simulink model "rst_auto_reg_teste"  (R2019a)
settings: Solver=VariableStepAuto  StartTime=0.0  StopTime=500  RelTol=1e-3
values from neighbouring files (symbols this model uses):
  A = den    [cod_teste_RST_4.m]
  B = num    [cod_teste_RST_4.m]
  ep = 0.9    [cod_teste_RST_4.m]
  R = [X(5) X(6) X(7) X(8)]    [cod_teste_RST_4.m]
  S = [X(1) X(2) X(3) X(4)]    [cod_teste_RST_4.m]
  T = sum(Am)/sum(B)    [cod_teste_RST_4.m]
  Ta = 0.1    [cod_teste_RST_4.m]
  Ts = 1    [cod_teste_RST_4.m]
undefined symbols (not defined in the file or in its folder): T_a
libraries: dspinverses x3
settings Model: Creator=Carlos Henrique  LastModifiedBy=PICHAU
settings DataIOCC: SaveOutput=off  SaveState=on  SignalLogging=off  DSMLogging=off  ReturnWorkspaceOutputs=off
settings DebuggingCC: ArithmeticOperatorsInVariantConditions=warning

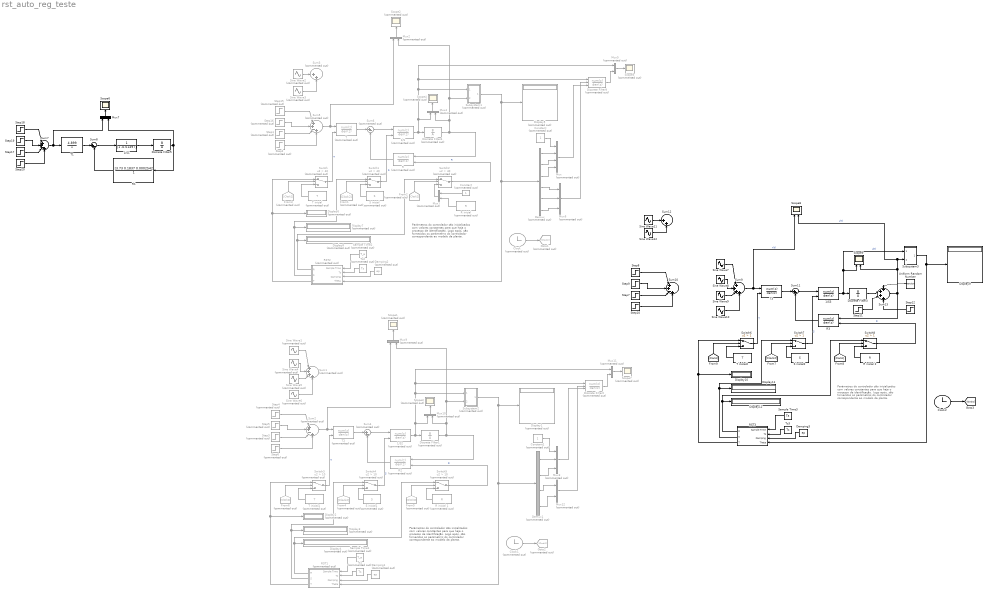
== system rst_auto_reg_teste ==
  note: Parâmetros do controlador são inicializados
      | com valores constantes para que haja o
      | processo de identificação. Logo após, são
      | fornecidos os parâmetros do controlador
      | correspondente ao modelo da planta.
  note: Parâmetros do controlador são inicializados
      | com valores constantes para que haja o
      | processo de identificação. Logo após, são
      | fornecidos os parâmetros do controlador
      | correspondente ao modelo da planta.
  note: Parâmetros do controlador são inicializados
      | com valores constantes para que haja o
      | processo de identificação. Logo após, são
      | fornecidos os parâmetros do controlador
      | correspondente ao modelo da planta.
  1/S : DiscreteFilter  Commented=on  Numerator=1  DenominatorSource=Input port  Denominator=1  a0EqualsOne=on
      settings: InputPortMap=u0,p3
  1/S1 : DiscreteFilter  Numerator=1  Denominator=[1 -0.01497]  a0EqualsOne=on
  1/S2 : DiscreteFilter  Commented=on  Numerator=1  DenominatorSource=Input port  Denominator=1  a0EqualsOne=on
      settings: InputPortMap=u0,p3
  1/S3 : DiscreteFilter  Numerator=1  DenominatorSource=Input port  Denominator=1  a0EqualsOne=on
      settings: InputPortMap=u0,p3
  Clock : Clock  Commented=on
  Clock1 : Clock  Commented=on
  Clock2 : Clock
  Constant : Constant  Commented=on
  "Constant " : Constant  Commented=on
  Constant1 : Constant  Commented=on
  Damping1 : Constant  Commented=on  Value=ep
  Damping2 : Constant  Commented=on  Value=ep
  Damping3 : Constant  Value=ep
  Demux : Demux  Commented=on  Outputs=6
  Demux1 : Demux  Commented=on
  Discrete Filter1 : DiscreteFilter  Commented=on  Numerator=B  Denominator=A  SampleTime=0.1  a0EqualsOne=on
  Discrete Filter2 : DiscreteFilter  Commented=on  NumeratorSource=Input port  Numerator=[3.317e-09 0.0355 0.02469]  DenominatorSource=Input port  Denominator=[1 -1.272 0.3317 0.0004192]  a0EqualsOne=on
      settings: InputPortMap=u0,p1,p3
  Discrete Filter3 : DiscreteFilter  Numerator=B  Denominator=A  SampleTime=0.1  a0EqualsOne=on
  Discrete Filter4 : DiscreteFilter  Commented=on  Numerator=B  Denominator=A  SampleTime=0.1  a0EqualsOne=on
  Discrete Filter5 : DiscreteFilter  Numerator=B  Denominator=A  SampleTime=0.1  a0EqualsOne=on
  Discrete Filter9 : DiscreteFilter  Commented=on  NumeratorSource=Input port  Numerator=[3.317e-09 0.0355 0.02469]  DenominatorSource=Input port  Denominator=[1 -1.272 0.3317 0.0004192]  a0EqualsOne=on
      settings: InputPortMap=u0,p1,p3
  Display{1..8} (8 alike) : Display  Commented=on
  Display{9..12} (4 alike) : Display
  From{1..6} (6 alike) : From  Commented=on  GotoTag=Clock2
  Goto1 : Goto  Commented=on  GotoTag=Clock2
  Goto2 : Goto  Commented=on  GotoTag=Clock2
  Mux : Mux  Commented=on
  Mux{1..2,4..5,9..12} (8 alike) : Mux  Commented=on  Inputs=2
  Mux3 : Mux  Commented=on  Inputs=3
  Mux6 : Mux  Commented=on  Inputs=3
  Mux7 : Mux  Inputs=2
  R : DiscreteFilter  Commented=on  NumeratorSource=Input port  Numerator=[-620.2 131.3]  Denominator=1
      settings: InputPortMap=u0,p1
  "R inicial " : Constant  Commented=on  Value=R
  R inicial 1 : Constant  Commented=on  Value=R
  R inicial 2 : Constant  Value=R
  R1 : DiscreteFilter  Numerator=[3.73 0.1837 0.0002542]  Denominator=1
  R2 : DiscreteFilter  Commented=on  NumeratorSource=Input port  Numerator=[-620.2 131.3]  Denominator=1
      settings: InputPortMap=u0,p1
  R3 : DiscreteFilter  NumeratorSource=Input port  Numerator=[-620.2 131.3]  Denominator=1
      settings: InputPortMap=u0,p1
  RST1 : Subsystem  Commented=on
  RST2 : Subsystem  Commented=on
  RST3 : Subsystem
  S inicial : Constant  Commented=on  Value=S
  S inicial1 : Constant  Commented=on  Value=S
  S inicial2 : Constant  Value=S
  Sample Time1 : Constant  Commented=on  Value=T_a
  Sample Time2 : Constant  Commented=on  Value=T_a
  Sample Time3 : Constant  Value=Ta
  Scope{1..5,7} (6 alike) : Scope  Commented=on
  Scope6 : Scope
  Scope8 : Scope  NumInputPorts=2
  Scope9 : Scope  NumInputPorts=2
  Sine Wave1 : Sin  Commented=on  SampleTime=0
  Sine Wave10 : Sin  Frequency=8  SampleTime=0
  Sine Wave11 : Sin  SampleTime=0
  Sine Wave12 : Sin  Frequency=2  SampleTime=0
  Sine Wave2 : Sin  Commented=on  SampleTime=0
  Sine Wave3 : Sin  Commented=on  Frequency=2  SampleTime=0
  Sine Wave4 : Sin  Commented=on  Frequency=2  SampleTime=0
  Sine Wave5 : Sin  Commented=on  Frequency=4  SampleTime=0
  Sine Wave6 : Sin  Commented=on  Frequency=8  SampleTime=0
  Sine Wave7 : Sin  SampleTime=0
  Sine Wave8 : Sin  Frequency=2  SampleTime=0
  Sine Wave9 : Sin  Frequency=4  SampleTime=0
  Step1 : Step  Commented=on  Time=20  After=2  SampleTime=0
  Step10 : Step  Time=30  SampleTime=0
  Step11 : Step  Time=50  SampleTime=0
  Step12 : Step  Time=51  After=-1  SampleTime=0
  Step15 : Step  Commented=on  Time=0  SampleTime=0
  Step16 : Step  Commented=on  Time=10  After=3  SampleTime=0
  Step17 : Step  Time=20  After=2  SampleTime=0
  Step18 : Step  Time=0  SampleTime=0
  Step19 : Step  Time=10  After=3  SampleTime=0
  Step2 : Step  Commented=on  Time=30  SampleTime=0
  Step20 : Step  Time=30  SampleTime=0
  Step3 : Step  Commented=on  Time=20  After=2  SampleTime=0
  Step4 : Step  Commented=on  Time=0  SampleTime=0
  Step5 : Step  Commented=on  Time=10  After=3  SampleTime=0
  Step6 : Step  Commented=on  Time=30  SampleTime=0
  Step7 : Step  Time=20  After=2  SampleTime=0
  Step8 : Step  Time=0  SampleTime=0
  Step9 : Step  Time=10  After=3  SampleTime=0
  Subsystem1 : Subsystem  Commented=on
  Subsystem2 : Subsystem  Commented=on
  Subsystem3 : Subsystem
  Sum1 : Sum  Commented=on  Inputs=|++++
  Sum10 : Sum  Inputs=|++-+
  Sum11 : Sum  Inputs=|+-
  Sum12 : Sum  Inputs=|++
  Sum13 : Sum  Inputs=++++
  Sum2 : Sum  Commented=on  Inputs=|++-+
  Sum3 : Sum  Commented=on  Inputs=|++
  Sum4 : Sum  Commented=on  Inputs=|+-
  Sum5 : Sum  Commented=on  Inputs=|++-+
  Sum6 : Sum  Commented=on  Inputs=|+-
  Sum7 : Sum  Inputs=|++-+
  Sum8 : Sum  Inputs=|+-
  Sum9 : Sum  Inputs=|++++
  Switch : Switch  Commented=on  Criteria=u2 > Threshold  Threshold=40
  Switch1 : Switch  Commented=on  Criteria=u2 > Threshold  Threshold=40
  Switch2 : Switch  Commented=on  Criteria=u2 > Threshold  Threshold=40
  Switch3 : Switch  Commented=on  Criteria=u2 > Threshold  Threshold=10
  Switch4 : Switch  Commented=on  Criteria=u2 > Threshold  Threshold=10
  Switch5 : Switch  Commented=on  Criteria=u2 > Threshold  Threshold=10
  Switch6 : Switch  Criteria=u2 > Threshold  Threshold=1
  Switch7 : Switch  Criteria=u2 > Threshold  Threshold=1
  Switch8 : Switch  Criteria=u2 > Threshold  Threshold=1
  T : DiscreteFilter  Commented=on  NumeratorSource=Input port  Numerator=13.39  Denominator=1
      settings: InputPortMap=u0,p1
  T inicial : Constant  Commented=on  Value=T
  T inicial1 : Constant  Commented=on  Value=T
  T inicial2 : Constant  Value=T
  T1 : DiscreteFilter  Numerator=4.899  Denominator=1  a0EqualsOne=on
  T2 : DiscreteFilter  Commented=on  NumeratorSource=Input port  Numerator=13.39  Denominator=1
      settings: InputPortMap=u0,p1
  T3 : DiscreteFilter  NumeratorSource=Input port  Numerator=13.39  Denominator=1
      settings: InputPortMap=u0,p1
  Ts1 : Constant  Commented=on  Value=Ts
  Ts2 : Constant  Commented=on  Value=Ts
  Ts3 : Constant  Value=Ts
  Uniform Random Number : UniformRandomNumber  Minimum=-0.1  Maximum=0.1  SampleTime=0
  wires:
  Sum6/1 -> 1/S/1
  R/1 -> Sum6/2
  Ts2/1 -> RST2/2(Ts)
  Step2/1 -> Sum5/4
  Damping2/1 -> RST2/3(Damping)
  Sum5/1 -> Mux2/1, T/1
  T/1 -> Sum6/1
  Step1/1 -> Sum5/3
  Step15/1 -> Sum5/1
  Step16/1 -> Sum5/2
  RST2/3(T) -> Switch/1, Display6/1
  Sample Time2/1 -> RST2/1(Sample Time)
  RST2/2(S) -> Switch1/1, Display7/1
  Mux5/1 -> Scope5/1
  Constant/1 -> Mux/1
  Demux/1 -> Mux/2
  Demux/2 -> Mux/3
  Demux/3 -> Mux/4
  Demux/4 -> Mux6/1
  Demux/5 -> Mux6/2
  Demux/6 -> Mux6/3
  Mux/1 -> Discrete Filter9/3
  Mux6/1 -> Discrete Filter9/2
  Discrete Filter9/1 -> Mux5/2
  1/S/1 -> Mux5/1, Discrete Filter9/1, Subsystem1/1(In1), Mux4/1, Discrete Filter4/1
  RST2/1(R) -> Switch2/1, Display8/1
  1/S1/1 -> Discrete Filter5/1
  Discrete Filter5/1 -> R1/1, Mux7/2
  Mux7/1 -> Scope6/1
  Step19/1 -> Sum7/2
  Step18/1 -> Sum7/1
  Step17/1 -> Sum7/3
  T1/1 -> Sum8/1
  Sum7/1 -> Mux7/1, T1/1
  Step20/1 -> Sum7/4
  R1/1 -> Sum8/2
  Sum8/1 -> 1/S1/1
  Discrete Filter4/1 -> R/1, Subsystem1/2(In2), Mux2/2, Mux4/2
  Mux4/1 -> Scope4/1
  T inicial/1 -> Switch/3
  From3/1 -> Switch/2
  Clock/1 -> Goto1/1
  Switch/1 -> T/2  "T"
  From1/1 -> Switch1/2
  Switch1/1 -> 1/S/2  "S"
  From2/1 -> Switch2/2
  Switch2/1 -> R/2  "R"
  S inicial/1 -> Switch1/3
  "R inicial "/1 -> Mux1/2
  "Constant "/1 -> Mux1/1
  Mux1/1 -> Switch2/3
  Subsystem1/1(Out1) -> RST2/4(Theta), Demux/1, Display5/1
  Mux2/1 -> Scope2/1
  Sine Wave2/1 -> Sum3/1
  Sine Wave3/1 -> Sum3/2
  Sine Wave4/1 -> Sum1/2
  Switch3/1 -> T2/2  "T"
  Mux9/1 -> Scope1/1
  Subsystem2/1(Out1) -> RST1/4(Theta), Demux1/1, Display1/1
  Switch4/1 -> 1/S2/2  "S"
  Switch5/1 -> R2/2  "R"
  Sum2/1 -> Mux9/1, T2/1
  Discrete Filter1/1 -> R2/1, Subsystem2/2(In2), Mux9/2, Mux10/2
  S inicial1/1 -> Switch4/3
  Sine Wave1/1 -> Sum1/1
  RST1/3(T) -> Switch3/1, Display2/1
  Damping1/1 -> RST1/3(Damping)
  T inicial1/1 -> Switch3/3
  From4/1 -> Switch4/2
  Sum4/1 -> 1/S2/1
  Mux10/1 -> Scope3/1
  Step5/1 -> Sum2/2
  Clock1/1 -> Goto2/1
  From6/1 -> Switch3/2
  From5/1 -> Switch5/2
  Demux1/1 -> Mux3/2
  Discrete Filter2/1 -> Mux11/2
  RST1/1(R) -> Switch5/1, Display4/1
  Mux3/1 -> Discrete Filter2/3
  1/S2/1 -> Mux11/1, Discrete Filter2/1, Subsystem2/1(In1), Mux10/1, Discrete Filter1/1
  Demux1/2 -> Mux3/3
  Mux11/1 -> Scope7/1
  Constant1/1 -> Mux3/1
  Step4/1 -> Sum2/1
  Mux12/1 -> Discrete Filter2/2
  Sample Time1/1 -> RST1/1(Sample Time)
  Step3/1 -> Sum2/3
  Step6/1 -> Sum2/4
  RST1/2(S) -> Switch4/1, Display3/1
  Ts1/1 -> RST1/2(Ts)
  R2/1 -> Sum4/2
  T2/1 -> Sum4/1
  Demux1/3 -> Mux12/1
  Demux1/4 -> Mux12/2
  R inicial 1/1 -> Switch5/3
  Sine Wave5/1 -> Sum1/3
  Sine Wave6/1 -> Sum1/4
  Sine Wave10/1 -> Sum9/4
  Ts3/1 -> RST3/2(Ts)
  T3/1 -> Sum11/1
  R3/1 -> Sum11/2
  RST3/1(R) -> Switch8/1, Display12/1
  Switch8/1 -> R3/2  "R"
  Step7/1 -> Sum10/3
  RST3/2(S) -> Switch7/1, Display11/1
  [Clock2] -> Switch7/2
  Sum13/1 -> R3/1, Scope9/2, Subsystem3/2(In2), Scope8/2  "y(t)"
  Subsystem3/1(Out1) -> RST3/4(Theta), Display9/1
  T inicial2/1 -> Switch6/3
  Sine Wave7/1 -> Sum9/1
  Clock2/1 -> [Clock2]
  S inicial2/1 -> Switch7/3
  Sum11/1 -> 1/S3/1
  Switch6/1 -> T3/2  "T"
  [Clock2] -> Switch6/2
  Switch7/1 -> 1/S3/2  "S"
  Sample Time3/1 -> RST3/1(Sample Time)
  Sine Wave8/1 -> Sum9/2
  Damping3/1 -> RST3/3(Damping)
  RST3/3(T) -> Switch6/1, Display10/1
  R inicial 2/1 -> Switch8/3
  Sine Wave9/1 -> Sum9/3
  Step9/1 -> Sum10/2
  Step8/1 -> Sum10/1
  Step10/1 -> Sum10/4
  1/S3/1 -> Scope9/1, Subsystem3/1(In1), Discrete Filter3/1  "u(t)"
  [Clock2] -> Switch8/2
  Sine Wave12/1 -> Sum12/2
  Sine Wave11/1 -> Sum12/1
  Discrete Filter3/1 -> Sum13/2
  Uniform Random Number/1 -> Sum13/1
  Step11/1 -> Sum13/3
  Step12/1 -> Sum13/4
  Sum9/1 -> Scope8/1, T3/1  "r(t)"

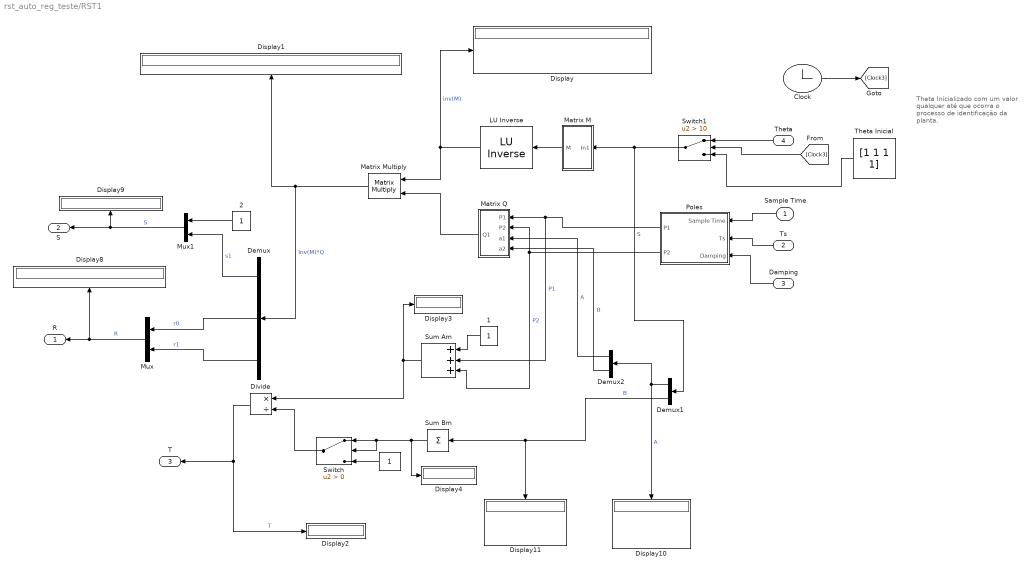
== system rst_auto_reg_teste/RST1 ==
  note: Theta Inicializado com um
      | valor qualquer até que ocorra
      |  o processo de identificação
      | da planta.
  Sample Time : Inport
  Ts : Inport  Port=2
  Damping : Inport  Port=3
  Theta : Inport  Port=4
  " " : Constant
  " LU Inverse" : dspinverses/ LU Inverse
      settings: SourceProductName=DSP System Toolbox
  1 : Constant
  2 : Constant
  Clock : Clock
  Demux : Demux  Outputs=3
  Demux1 : Demux  Outputs=2
  Demux2 : Demux  Outputs=2
  Display{,1..4,8..11} (9 alike) : Display
  Divide : Product  Inputs=*/
  Matrix M : Subsystem
  Matrix Multiply : Product  Multiplication=Matrix(*)
  Matrix Q : Subsystem
  Mux : Mux  Inputs=2
  Mux1 : Mux  Inputs=2
  Poles : Subsystem
  Sum Am : Sum  Inputs=+++
  Sum Bm : Sum  Inputs=+
  Switch : Switch  Criteria=u2 > Threshold
  Switch1 : Switch  Criteria=u2 > Threshold  Threshold=10
  Theta Inicial : Constant  Value=[1 1 1 1]
  R : Outport
  S : Outport  Port=2
  T : Outport  Port=3
  wires:
  Matrix Multiply/1 -> Demux/1, Display1/1  "Inv(M)*Q"
  Sum Bm/1 -> Switch/2, Switch/1, Display4/1
  " LU Inverse"/1 -> Matrix Multiply/1, Display/1  "inv(M)"
  Sum Am/1 -> Divide/1, Display3/1
  Mux1/1 -> S/1, Display9/1  "S"
  Poles/2(P2) -> Sum Am/3, Matrix Q/2(P2)  "P2"
  Divide/1 -> T/1, Display2/1  "T"
  Ts/1 -> Poles/2(Ts)
  Damping/1 -> Poles/3(Damping)
  Sample Time/1 -> Poles/1(Sample Time)
  1/1 -> Sum Am/1
  Poles/1(P1) -> Sum Am/2, Matrix Q/1(P1)  "P1"
  Demux1/2 -> Display11/1, Sum Bm/1  "B"
  Demux1/1 -> Display10/1, Demux2/1  "A"
  Switch/1 -> Divide/2
  " "/1 -> Switch/3
  Mux/1 -> R/1, Display8/1  "R"
  Clock/1 -> [Clock3]
  Switch1/1 -> Matrix M/1(In1), Demux1/1  "S"
  Theta/1 -> Switch1/1
  [Clock3] -> Switch1/2
  Theta Inicial/1 -> Switch1/3
  Matrix M/1(M) -> " LU Inverse"/1
  Matrix Q/1(Q1) -> Matrix Multiply/2
  Demux2/1 -> Matrix Q/3(a1)  "A"
  Demux2/2 -> Matrix Q/4(a2)  "B"
  Demux/2 -> Mux/1  "r0"
  Demux/3 -> Mux/2  "r1"
  Demux/1 -> Mux1/2  "s1"
  2/1 -> Mux1/1

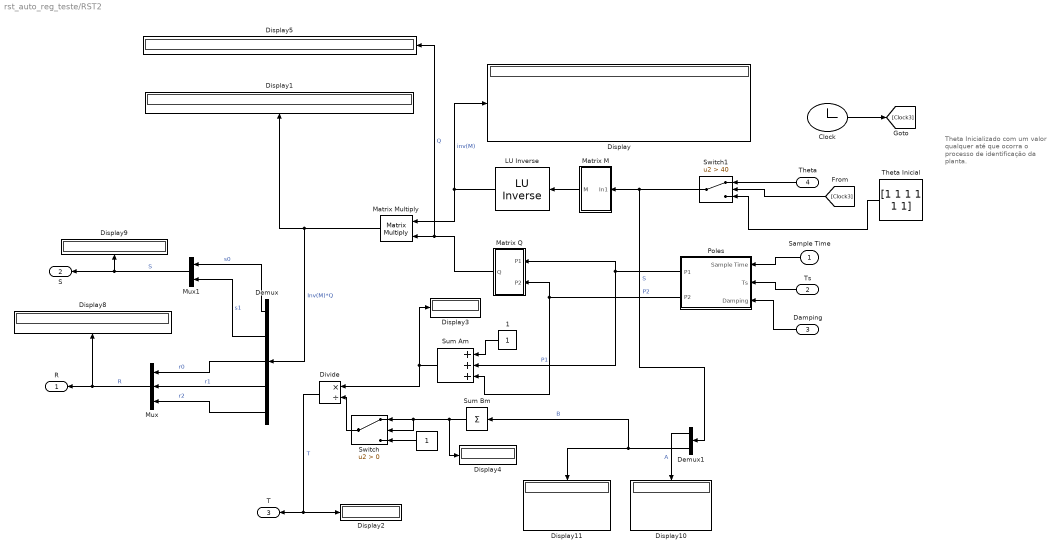
== system rst_auto_reg_teste/RST2 ==
  note: Theta Inicializado com um
      | valor qualquer até que ocorra
      |  o processo de identificação
      | da planta.
  Sample Time : Inport
  Ts : Inport  Port=2
  Damping : Inport  Port=3
  Theta : Inport  Port=4
  " " : Constant
  " LU Inverse" : dspinverses/ LU Inverse
      settings: SourceProductName=DSP System Toolbox
  1 : Constant
  Clock : Clock
  Demux : Demux  Outputs=5
  Demux1 : Demux  Outputs=2
  Display{,1..5,8..11} (10 alike) : Display
  Divide : Product  Inputs=*/
  Matrix M : Subsystem
  Matrix Multiply : Product  Multiplication=Matrix(*)
  Matrix Q : Subsystem
  Mux : Mux  Inputs=3
  Mux1 : Mux  Inputs=2
  Poles : Subsystem
  Sum Am : Sum  Inputs=+++
  Sum Bm : Sum  Inputs=+
  Switch : Switch  Criteria=u2 > Threshold
  Switch1 : Switch  Criteria=u2 > Threshold  Threshold=40
  Theta Inicial : Constant  Value=[1 1 1 1 1 1]
  R : Outport
  S : Outport  Port=2
  T : Outport  Port=3
  wires:
  Matrix Multiply/1 -> Demux/1, Display1/1  "Inv(M)*Q"
  Sum Bm/1 -> Switch/2, Switch/1, Display4/1
  " LU Inverse"/1 -> Matrix Multiply/1, Display/1  "inv(M)"
  Sum Am/1 -> Divide/1, Display3/1
  Mux1/1 -> S/1, Display9/1  "S"
  Poles/2(P2) -> Matrix Q/2(P2), Sum Am/3  "P2"
  Divide/1 -> T/1, Display2/1  "T"
  Ts/1 -> Poles/2(Ts)
  Matrix Q/1(Q) -> Display5/1, Matrix Multiply/2  "Q"
  Damping/1 -> Poles/3(Damping)
  Sample Time/1 -> Poles/1(Sample Time)
  1/1 -> Sum Am/1
  Matrix M/1(M) -> " LU Inverse"/1
  Poles/1(P1) -> Sum Am/2, Matrix Q/1(P1)  "P1"
  Demux1/2 -> Sum Bm/1, Display11/1  "B"
  Demux1/1 -> Display10/1  "A"
  Switch/1 -> Divide/2
  " "/1 -> Switch/3
  Demux/1 -> Mux1/1  "s0"
  Demux/2 -> Mux1/2  "s1"
  Mux/1 -> R/1, Display8/1  "R"
  Demux/3 -> Mux/1  "r0"
  Demux/4 -> Mux/2  "r1"
  Demux/5 -> Mux/3  "r2"
  Clock/1 -> [Clock3]
  Switch1/1 -> Demux1/1, Matrix M/1(In1)  "S"
  Theta/1 -> Switch1/1
  [Clock3] -> Switch1/2
  Theta Inicial/1 -> Switch1/3

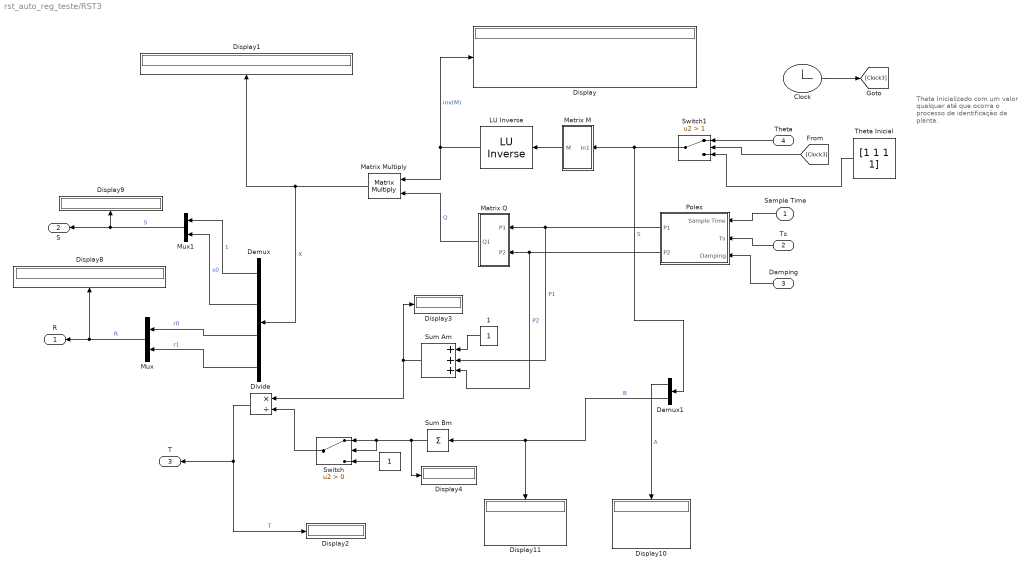
== system rst_auto_reg_teste/RST3 ==
  note: Theta Inicializado com um
      | valor qualquer até que ocorra
      |  o processo de identificação
      | da planta.
  Sample Time : Inport
  Ts : Inport  Port=2
  Damping : Inport  Port=3
  Theta : Inport  Port=4
  " " : Constant
  " LU Inverse" : dspinverses/ LU Inverse
      settings: SourceProductName=DSP System Toolbox
  1 : Constant
  Clock : Clock
  Demux : Demux
  Demux1 : Demux  Outputs=2
  Display{,1..4,8..11} (9 alike) : Display
  Divide : Product  Inputs=*/
  Matrix M : Subsystem
  Matrix Multiply : Product  Multiplication=Matrix(*)
  Matrix Q : Subsystem
  Mux : Mux  Inputs=2
  Mux1 : Mux  Inputs=2
  Poles : Subsystem
  Sum Am : Sum  Inputs=+++
  Sum Bm : Sum  Inputs=+
  Switch : Switch  Criteria=u2 > Threshold
  Switch1 : Switch  Criteria=u2 > Threshold  Threshold=1
  Theta Inicial : Constant  Value=[1 1 1 1]
  R : Outport
  S : Outport  Port=2
  T : Outport  Port=3
  wires:
  Matrix Multiply/1 -> Demux/1, Display1/1  "X"
  Sum Bm/1 -> Switch/2, Switch/1, Display4/1
  " LU Inverse"/1 -> Matrix Multiply/1, Display/1  "inv(M)"
  Sum Am/1 -> Divide/1, Display3/1
  Mux1/1 -> S/1, Display9/1  "S"
  Poles/2(P2) -> Matrix Q/2(P2), Sum Am/3  "P2"
  Divide/1 -> T/1, Display2/1  "T"
  Ts/1 -> Poles/2(Ts)
  Damping/1 -> Poles/3(Damping)
  Sample Time/1 -> Poles/1(Sample Time)
  1/1 -> Sum Am/1
  Poles/1(P1) -> Matrix Q/1(P1), Sum Am/2  "P1"
  Demux1/2 -> Display11/1, Sum Bm/1  "B"
  Demux1/1 -> Display10/1  "A"
  Switch/1 -> Divide/2
  " "/1 -> Switch/3
  Mux/1 -> R/1, Display8/1  "R"
  Clock/1 -> [Clock3]
  Switch1/1 -> Matrix M/1(In1), Demux1/1  "S"
  Theta/1 -> Switch1/1
  [Clock3] -> Switch1/2
  Theta Inicial/1 -> Switch1/3
  Matrix M/1(M) -> " LU Inverse"/1
  Matrix Q/1(Q1) -> Matrix Multiply/2  "Q"
  Demux/1 -> Mux1/1  "1"
  Demux/2 -> Mux1/2  "s0"
  Demux/3 -> Mux/1  "r0"
  Demux/4 -> Mux/2  "r1"

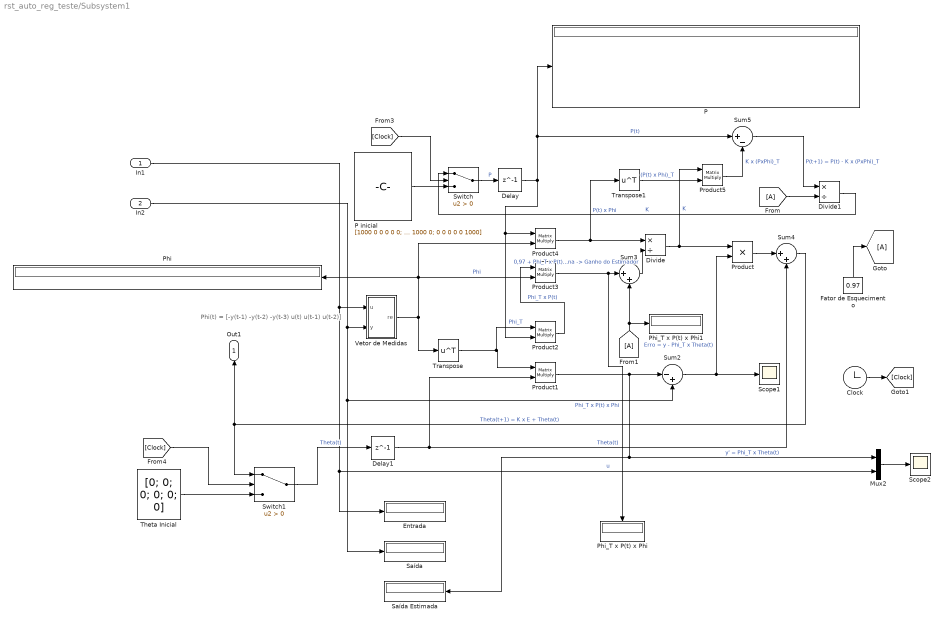
== system rst_auto_reg_teste/Subsystem1 ==
  note: Phi(t) = [-y(t-1) -y(t-2) -y(t-3) u(t) u(t-1) u(t-2)]
  In1 : Inport
  In2 : Inport  Port=2
  Clock : Clock
  Delay : Delay  DelayLength=1  InitialCondition=0  SampleTime=0.1
  Delay1 : Delay  DelayLength=1  InitialCondition=0  SampleTime=0.1
  Divide : Product  Inputs=*/
  Divide1 : Product  Inputs=*/
  Entrada : Display
  "Fator de Esquecimento " : Constant  Value=0.97
  Mux2 : Mux  Inputs=2
  P : Display
  P inicial : Constant  Value=[1000 0 0 0 0 0; 0 1000 0 0 0 0; 0 0 1000 0 0 0; 0 0 0 1000 0 0; 0 0 0 0 1000 0; 0 0 0 0 0 1000]
  Phi : Display
  Phi_T x P(t) x Phi : Display
  Phi_T x P(t) x Phi1 : Display
  Product : Product
  Product{1..5} (5 alike) : Product  Multiplication=Matrix(*)
  Saída : Display
  "Saída Estimada " : Display
  Scope1 : Scope
  Scope2 : Scope
  Sum2 : Sum  Inputs=|-+
  Sum3 : Sum  Inputs=|++
  Sum4 : Sum  Inputs=|++
  Sum5 : Sum  Inputs=|+-
  Switch : Switch  Criteria=u2 > Threshold
  Switch1 : Switch  Criteria=u2 > Threshold
  "Theta Inicial " : Constant  Value=[0; 0; 0; 0; 0; 0]
  Transpose : Math  Operator=transpose  SaturateOnIntegerOverflow=on
  Transpose1 : Math  Operator=transpose  SaturateOnIntegerOverflow=on
  "Vetor de Medidas " : Subsystem
  Out1 : Outport
  wires:
  "Vetor de Medidas "/1(re) -> Product4/2, Phi/1, Product3/2, Transpose/1  "Phi"
  Product/1 -> Sum4/1
  In2/1 -> Saída/1, Sum2/2, "Vetor de Medidas "/2(y)
  "Fator de Esquecimento "/1 -> [A]
  Transpose/1 -> Product2/1, Product1/1  "Phi_T"
  Sum3/1 -> Divide/2  "0,97 + Phi_T x P(t) x Phi Vetor Coluna -> Ganho do Estimador"
  Product3/1 -> Phi_T x P(t) x Phi/1, Sum3/1  "Phi_T x P(t) x Phi"
  Switch/1 -> Delay/1  "P"
  Product4/1 -> Transpose1/1, Divide/1  "P(t) x Phi"
  Delay/1 -> Product2/2, Product4/1, P/1, Sum5/1  "P(t)"
  Divide/1 -> Product5/1, Product/1  "K"
  Transpose1/1 -> Product5/2  "(P(t) x Phi)_T"
  Sum5/1 -> Divide1/1  "P(t+1) = P(t) - K x (PxPhi)_T"
  Sum2/1 -> Scope1/1, Product/2  "Erro = y - Phi_T x Theta(t)"
  Delay1/1 -> Sum4/2, Product1/2  "Theta(t)"
  Divide1/1 -> Switch/1  "K"
  "Theta Inicial "/1 -> Switch1/3
  [A] -> Divide1/2
  Product2/1 -> Product3/1  "Phi_T x P(t)"
  Clock/1 -> [Clock]
  Product1/1 -> Mux2/1, "Saída Estimada "/1, Sum2/1  "y' = Phi_T x Theta(t)"
  Product5/1 -> Sum5/2  "K x (PxPhi)_T"
  P inicial/1 -> Switch/3
  Sum4/1 -> Switch1/1, Out1/1  "Theta(t+1) = K x E + Theta(t)"
  [A] -> Sum3/2, Phi_T x P(t) x Phi1/1
  In1/1 -> Entrada/1, Mux2/2, "Vetor de Medidas "/1(u)  "u"
  [Clock] -> Switch/2
  Switch1/1 -> Delay1/1  "Theta(t)"
  Mux2/1 -> Scope2/1
  [Clock] -> Switch1/2

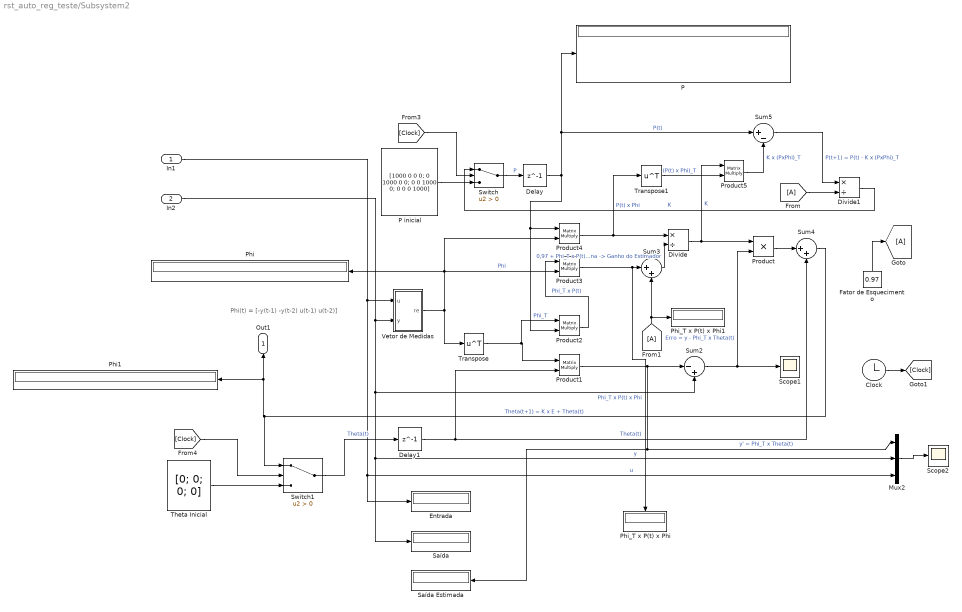
== system rst_auto_reg_teste/Subsystem2 ==
  note: Phi(t) = [-y(t-1) -y(t-2) u(t-1) u(t-2)]
  In1 : Inport
  In2 : Inport  Port=2
  Clock : Clock
  Delay : Delay  DelayLength=1  InitialCondition=0  SampleTime=0.1
  Delay1 : Delay  DelayLength=1  InitialCondition=0  SampleTime=0.1
  Divide : Product  Inputs=*/
  Divide1 : Product  Inputs=*/
  Entrada : Display
  "Fator de Esquecimento " : Constant  Value=0.97
  Mux2 : Mux  Inputs=3
  P : Display
  P inicial : Constant  Value=[1000 0 0 0; 0 1000 0 0; 0 0 1000 0; 0 0 0 1000]
  Phi : Display
  Phi1 : Display
  Phi_T x P(t) x Phi : Display
  Phi_T x P(t) x Phi1 : Display
  Product : Product
  Product{1..5} (5 alike) : Product  Multiplication=Matrix(*)
  Saída : Display
  "Saída Estimada " : Display
  Scope1 : Scope
  Scope2 : Scope
  Sum2 : Sum  Inputs=|-+
  Sum3 : Sum  Inputs=|++
  Sum4 : Sum  Inputs=|++
  Sum5 : Sum  Inputs=|+-
  Switch : Switch  Criteria=u2 > Threshold
  Switch1 : Switch  Criteria=u2 > Threshold
  "Theta Inicial " : Constant  Value=[0; 0; 0; 0]
  Transpose : Math  Operator=transpose  SaturateOnIntegerOverflow=on
  Transpose1 : Math  Operator=transpose  SaturateOnIntegerOverflow=on
  "Vetor de Medidas " : Subsystem
  Out1 : Outport
  wires:
  "Vetor de Medidas "/1(re) -> Product4/2, Phi/1, Product3/2, Transpose/1  "Phi"
  Product/1 -> Sum4/1
  In2/1 -> Mux2/2, Saída/1, Sum2/2, "Vetor de Medidas "/2(y)  "y"
  "Fator de Esquecimento "/1 -> [A]
  Transpose/1 -> Product2/1, Product1/1  "Phi_T"
  Sum3/1 -> Divide/2  "0,97 + Phi_T x P(t) x Phi Vetor Coluna -> Ganho do Estimador"
  Product3/1 -> Phi_T x P(t) x Phi/1, Sum3/1  "Phi_T x P(t) x Phi"
  Switch/1 -> Delay/1  "P"
  Product4/1 -> Transpose1/1, Divide/1  "P(t) x Phi"
  Delay/1 -> Product2/2, Product4/1, P/1, Sum5/1  "P(t)"
  Divide/1 -> Product5/1, Product/1  "K"
  Transpose1/1 -> Product5/2  "(P(t) x Phi)_T"
  Sum5/1 -> Divide1/1  "P(t+1) = P(t) - K x (PxPhi)_T"
  Sum2/1 -> Scope1/1, Product/2  "Erro = y - Phi_T x Theta(t)"
  Delay1/1 -> Sum4/2, Product1/2  "Theta(t)"
  Divide1/1 -> Switch/1  "K"
  "Theta Inicial "/1 -> Switch1/3
  [A] -> Divide1/2
  Product2/1 -> Product3/1  "Phi_T x P(t)"
  Clock/1 -> [Clock]
  Product1/1 -> Sum2/1, Mux2/1, "Saída Estimada "/1  "y' = Phi_T x Theta(t)"
  Product5/1 -> Sum5/2  "K x (PxPhi)_T"
  P inicial/1 -> Switch/3
  Sum4/1 -> Switch1/1, Phi1/1, Out1/1  "Theta(t+1) = K x E + Theta(t)"
  [A] -> Sum3/2, Phi_T x P(t) x Phi1/1
  In1/1 -> Mux2/3, Entrada/1, "Vetor de Medidas "/1(u)  "u"
  [Clock] -> Switch/2
  Switch1/1 -> Delay1/1  "Theta(t)"
  Mux2/1 -> Scope2/1
  [Clock] -> Switch1/2

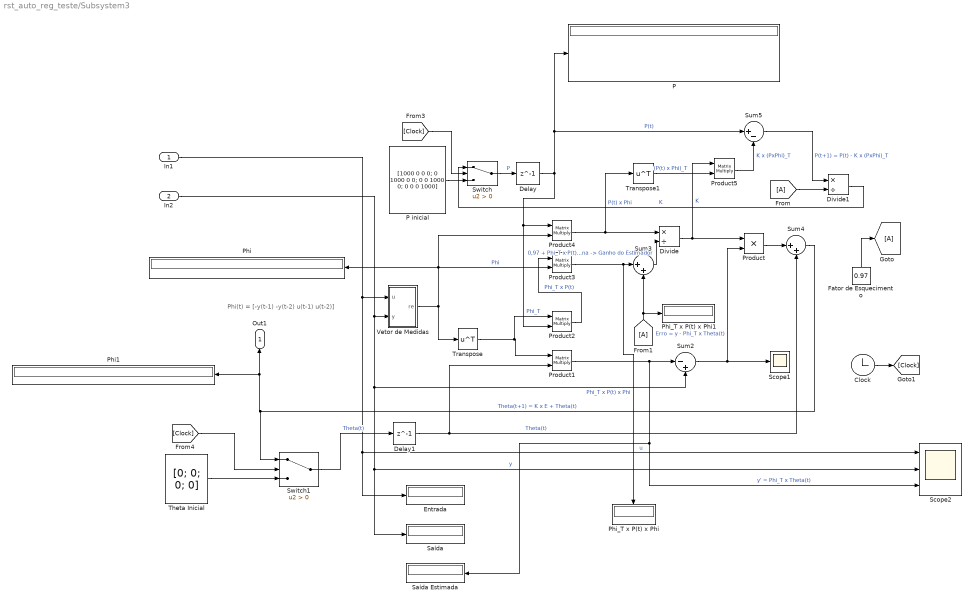
== system rst_auto_reg_teste/Subsystem3 ==
  note: Phi(t) = [-y(t-1) -y(t-2) u(t-1) u(t-2)]
  In1 : Inport
  In2 : Inport  Port=2
  Clock : Clock
  Delay : Delay  DelayLength=1  InitialCondition=0  SampleTime=0.1
  Delay1 : Delay  DelayLength=1  InitialCondition=0  SampleTime=0.1
  Divide : Product  Inputs=*/
  Divide1 : Product  Inputs=*/
  Entrada : Display
  "Fator de Esquecimento " : Constant  Value=0.97
  P : Display
  P inicial : Constant  Value=[1000 0 0 0; 0 1000 0 0; 0 0 1000 0; 0 0 0 1000]
  Phi : Display
  Phi1 : Display
  Phi_T x P(t) x Phi : Display
  Phi_T x P(t) x Phi1 : Display
  Product : Product
  Product{1..5} (5 alike) : Product  Multiplication=Matrix(*)
  Saída : Display
  "Saída Estimada " : Display
  Scope1 : Scope
  Scope2 : Scope  NumInputPorts=3
  Sum2 : Sum  Inputs=|-+
  Sum3 : Sum  Inputs=|++
  Sum4 : Sum  Inputs=|++
  Sum5 : Sum  Inputs=|+-
  Switch : Switch  Criteria=u2 > Threshold
  Switch1 : Switch  Criteria=u2 > Threshold
  "Theta Inicial " : Constant  Value=[0; 0; 0; 0]
  Transpose : Math  Operator=transpose  SaturateOnIntegerOverflow=on
  Transpose1 : Math  Operator=transpose  SaturateOnIntegerOverflow=on
  "Vetor de Medidas " : Subsystem
  Out1 : Outport
  wires:
  "Vetor de Medidas "/1(re) -> Product4/2, Phi/1, Product3/2, Transpose/1  "Phi"
  Product/1 -> Sum4/1
  In2/1 -> Saída/1, Scope2/2, Sum2/2, "Vetor de Medidas "/2(y)  "y"
  "Fator de Esquecimento "/1 -> [A]
  Transpose/1 -> Product2/1, Product1/1  "Phi_T"
  Sum3/1 -> Divide/2  "0,97 + Phi_T x P(t) x Phi Vetor Coluna -> Ganho do Estimador"
  Product3/1 -> Phi_T x P(t) x Phi/1, Sum3/1  "Phi_T x P(t) x Phi"
  Switch/1 -> Delay/1  "P"
  Product4/1 -> Transpose1/1, Divide/1  "P(t) x Phi"
  Delay/1 -> Product2/2, Product4/1, P/1, Sum5/1  "P(t)"
  Divide/1 -> Product5/1, Product/1  "K"
  Transpose1/1 -> Product5/2  "(P(t) x Phi)_T"
  Sum5/1 -> Divide1/1  "P(t+1) = P(t) - K x (PxPhi)_T"
  Sum2/1 -> Scope1/1, Product/2  "Erro = y - Phi_T x Theta(t)"
  Delay1/1 -> Sum4/2, Product1/2  "Theta(t)"
  Divide1/1 -> Switch/1  "K"
  "Theta Inicial "/1 -> Switch1/3
  [A] -> Divide1/2
  Product2/1 -> Product3/1  "Phi_T x P(t)"
  Clock/1 -> [Clock]
  Product1/1 -> Sum2/1, Scope2/3, "Saída Estimada "/1  "y' = Phi_T x Theta(t)"
  Product5/1 -> Sum5/2  "K x (PxPhi)_T"
  P inicial/1 -> Switch/3
  Sum4/1 -> Switch1/1, Phi1/1, Out1/1  "Theta(t+1) = K x E + Theta(t)"
  [A] -> Sum3/2, Phi_T x P(t) x Phi1/1
  In1/1 -> Entrada/1, Scope2/1, "Vetor de Medidas "/1(u)  "u"
  [Clock] -> Switch/2
  Switch1/1 -> Delay1/1  "Theta(t)"
  [Clock] -> Switch1/2

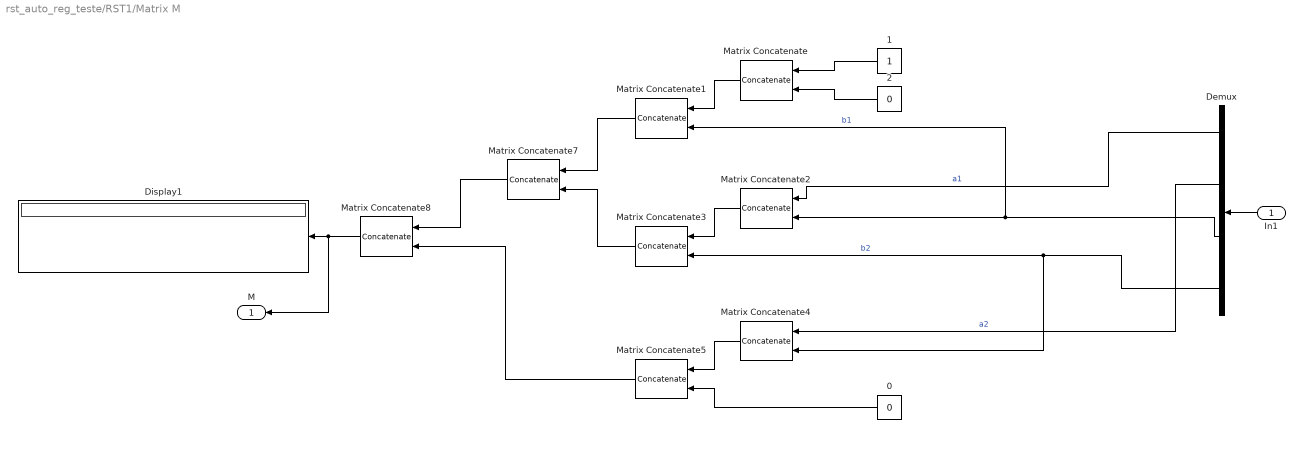
== system rst_auto_reg_teste/RST1/Matrix M ==
  In1 : Inport
  " 0" : Constant  Value=0
  " 2" : Constant  Value=0
  1 : Constant
  Demux : Demux
  Display1 : Display
  Matrix Concatenate{,1..5} (6 alike) : Concatenate  Mode=Multidimensional array  ConcatenateDimension=2
  Matrix Concatenate7 : Concatenate  Mode=Multidimensional array
  Matrix Concatenate8 : Concatenate  Mode=Multidimensional array
  M : Outport
  wires:
  In1/1 -> Demux/1
  1/1 -> Matrix Concatenate/1
  Matrix Concatenate5/1 -> Matrix Concatenate8/2
  Matrix Concatenate4/1 -> Matrix Concatenate5/1
  " 2"/1 -> Matrix Concatenate/2
  Demux/3 -> Matrix Concatenate1/2, Matrix Concatenate2/2  "b1"
  Matrix Concatenate2/1 -> Matrix Concatenate3/1
  Matrix Concatenate1/1 -> Matrix Concatenate7/1
  Matrix Concatenate3/1 -> Matrix Concatenate7/2
  " 0"/1 -> Matrix Concatenate5/2
  Matrix Concatenate7/1 -> Matrix Concatenate8/1
  Matrix Concatenate/1 -> Matrix Concatenate1/1
  Matrix Concatenate8/1 -> M/1, Display1/1
  Demux/1 -> Matrix Concatenate2/1  "a1"
  Demux/4 -> Matrix Concatenate4/2, Matrix Concatenate3/2  "b2"
  Demux/2 -> Matrix Concatenate4/1  "a2"

== system rst_auto_reg_teste/RST1/Matrix Q ==
  P1 : Inport
  P2 : Inport  Port=2
  a1 : Inport  Port=3
  a2 : Inport  Port=4
  2 : Constant  Value=0
  Display1 : Display
  Matrix Concatenate1 : Concatenate  Mode=Multidimensional array
  Matrix Concatenate2 : Concatenate  Mode=Multidimensional array
  Subtract : Sum  Inputs=+-
  Subtract1 : Sum  Inputs=+-
  Q1 : Outport
  wires:
  Subtract/1 -> Matrix Concatenate1/1
  P2/1 -> Subtract1/1
  Matrix Concatenate1/1 -> Matrix Concatenate2/1
  Matrix Concatenate2/1 -> Q1/1, Display1/1
  2/1 -> Matrix Concatenate2/2
  P1/1 -> Subtract/1
  Subtract1/1 -> Matrix Concatenate1/2
  a2/1 -> Subtract1/2
  a1/1 -> Subtract/2

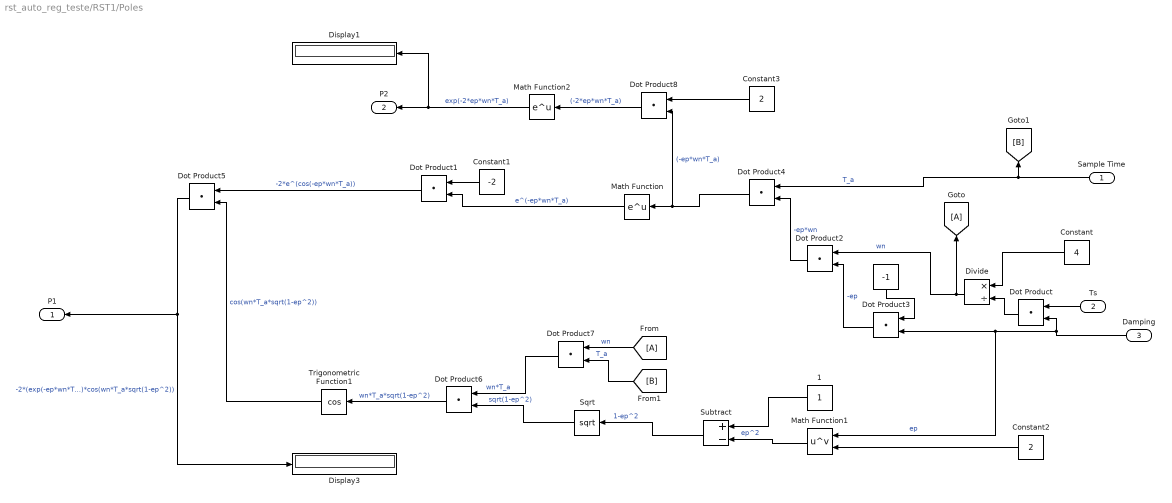
== system rst_auto_reg_teste/RST1/Poles ==
  Sample Time : Inport
  Ts : Inport  Port=2
  Damping : Inport  Port=3
  " " : Constant  Value=-1
  1 : Constant
  Constant : Constant  Value=4
  Constant1 : Constant  Value=-2
  Constant2 : Constant  Value=2
  Constant3 : Constant  Value=2
  Display1 : Display
  Display3 : Display
  Divide : Product  Inputs=*/
  Dot Product{,1..8} (9 alike) : DotProduct  InputSameDT=on  OutDataTypeStr=Inherit: Inherit via internal rule
  Math Function : Math  SaturateOnIntegerOverflow=on
  Math Function1 : Math  Operator=pow  SaturateOnIntegerOverflow=on
  Math Function2 : Math  SaturateOnIntegerOverflow=on
  Sqrt : Sqrt  SaturateOnIntegerOverflow=on
  Subtract : Sum  Inputs=+-
  Trigonometric Function1 : Trigonometry  Operator=cos
  P1 : Outport
  P2 : Outport  Port=2
  wires:
  Math Function/1 -> Dot Product1/2  "e^(-ep*wn*T_a)"
  Divide/1 -> [A], Dot Product2/1  "wn"
  [A] -> Dot Product7/1  "wn"
  " "/1 -> Dot Product3/1
  Dot Product5/1 -> P1/1, Display3/1  "-2*(exp(-ep*wn*T_a))*cos(wn*T_a*sqrt(1-ep^2))"
  Trigonometric Function1/1 -> Dot Product5/2  "cos(wn*T_a*sqrt(1-ep^2))"
  Ts/1 -> Dot Product/1
  Dot Product/1 -> Divide/2
  Dot Product3/1 -> Dot Product2/2  "-ep"
  Damping/1 -> Math Function1/1, Dot Product3/2, Dot Product/2  "ep"
  Constant/1 -> Divide/1
  Dot Product7/1 -> Dot Product6/1  "wn*T_a"
  Sample Time/1 -> Dot Product4/1, [B]  "T_a"
  Math Function1/1 -> Subtract/2  "ep^2"
  Dot Product1/1 -> Dot Product5/1  "-2*e^(cos(-ep*wn*T_a))"
  Constant2/1 -> Math Function1/2
  1/1 -> Subtract/1
  Constant1/1 -> Dot Product1/1
  Dot Product2/1 -> Dot Product4/2  "-ep*wn"
  [B] -> Dot Product7/2  "T_a"
  Dot Product6/1 -> Trigonometric Function1/1  "wn*T_a*sqrt(1-ep^2)"
  Dot Product4/1 -> Dot Product8/2, Math Function/1  "(-ep*wn*T_a)"
  Sqrt/1 -> Dot Product6/2  "sqrt(1-ep^2)"
  Subtract/1 -> Sqrt/1  "1-ep^2"
  Constant3/1 -> Dot Product8/1
  Dot Product8/1 -> Math Function2/1  "(-2*ep*wn*T_a)"
  Math Function2/1 -> Display1/1, P2/1  "exp(-2*ep*wn*T_a)"

== system rst_auto_reg_teste/RST2/Matrix M ==
  In1 : Inport
  " " : Constant  Value=0
  " 1" : Constant
  Demux : Demux  Outputs=6
  Display : Display
  Matrix Concatenate{,1..4} (5 alike) : Concatenate  NumInputs=5  Mode=Multidimensional array  ConcatenateDimension=2
  Matrix Concatenate6 : Concatenate  NumInputs=5  Mode=Multidimensional array
  M : Outport
  wires:
  In1/1 -> Demux/1
  Matrix Concatenate6/1 -> M/1, Display/1
  Matrix Concatenate/1 -> Matrix Concatenate6/1
  Matrix Concatenate2/1 -> Matrix Concatenate6/2
  Matrix Concatenate1/1 -> Matrix Concatenate6/3
  Matrix Concatenate3/1 -> Matrix Concatenate6/4
  " 1"/1 -> Matrix Concatenate2/2, Matrix Concatenate/1
  " "/1 -> Matrix Concatenate4/4, Matrix Concatenate4/3, Matrix Concatenate4/1, Matrix Concatenate3/3, Matrix Concatenate2/5, Matrix Concatenate/5, Matrix Concatenate/4, Matrix Concatenate/2
  Demux/4 -> Matrix Concatenate2/4, Matrix Concatenate/3, Matrix Concatenate1/5  "b0"
  Demux/1 -> Matrix Concatenate1/2, Matrix Concatenate2/1  "a1"
  Demux/5 -> Matrix Concatenate3/5, Matrix Concatenate1/4, Matrix Concatenate2/3  "b1"
  Demux/2 -> Matrix Concatenate3/2, Matrix Concatenate1/1  "a2"
  Demux/6 -> Matrix Concatenate4/5, Matrix Concatenate3/4, Matrix Concatenate1/3  "b2"
  Demux/3 -> Matrix Concatenate3/1, Matrix Concatenate4/2  "a3"
  Matrix Concatenate4/1 -> Matrix Concatenate6/5

== system rst_auto_reg_teste/RST2/Matrix Q ==
  P1 : Inport
  P2 : Inport  Port=2
  0 : Constant  Value=0
  1 : Constant
  Display : Display
  Matrix Concatenate : Concatenate  NumInputs=5  Mode=Multidimensional array
  Q : Outport
  wires:
  Matrix Concatenate/1 -> Q/1, Display/1
  1/1 -> Matrix Concatenate/1
  P1/1 -> Matrix Concatenate/2
  P2/1 -> Matrix Concatenate/3
  0/1 -> Matrix Concatenate/5, Matrix Concatenate/4

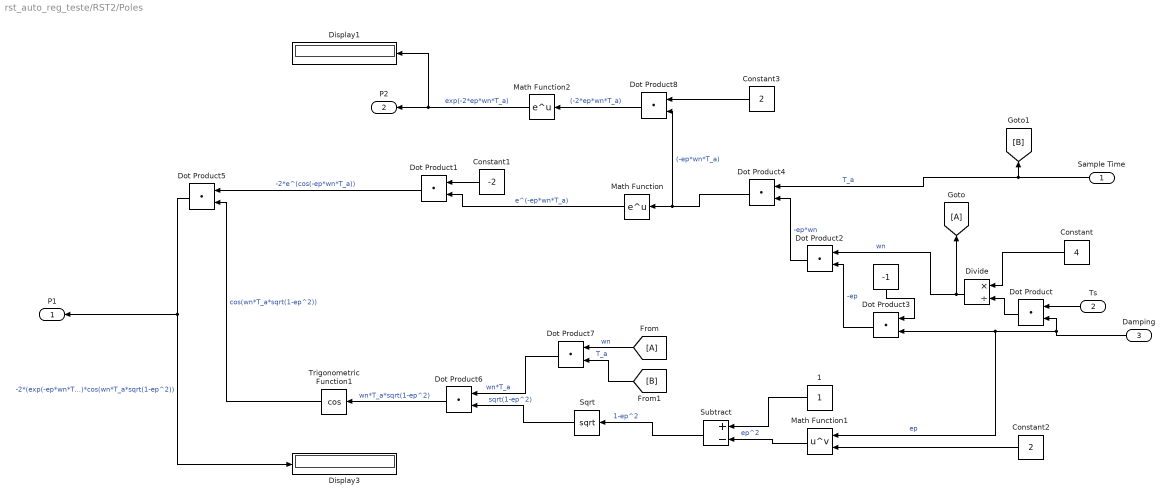
== system rst_auto_reg_teste/RST2/Poles ==
  Sample Time : Inport
  Ts : Inport  Port=2
  Damping : Inport  Port=3
  " " : Constant  Value=-1
  1 : Constant
  Constant : Constant  Value=4
  Constant1 : Constant  Value=-2
  Constant2 : Constant  Value=2
  Constant3 : Constant  Value=2
  Display1 : Display
  Display3 : Display
  Divide : Product  Inputs=*/
  Dot Product{,1..8} (9 alike) : DotProduct  InputSameDT=on  OutDataTypeStr=Inherit: Inherit via internal rule
  Math Function : Math  SaturateOnIntegerOverflow=on
  Math Function1 : Math  Operator=pow  SaturateOnIntegerOverflow=on
  Math Function2 : Math  SaturateOnIntegerOverflow=on
  Sqrt : Sqrt  SaturateOnIntegerOverflow=on
  Subtract : Sum  Inputs=+-
  Trigonometric Function1 : Trigonometry  Operator=cos
  P1 : Outport
  P2 : Outport  Port=2
  wires:
  Math Function/1 -> Dot Product1/2  "e^(-ep*wn*T_a)"
  Divide/1 -> [A], Dot Product2/1  "wn"
  [A] -> Dot Product7/1  "wn"
  " "/1 -> Dot Product3/1
  Dot Product5/1 -> P1/1, Display3/1  "-2*(exp(-ep*wn*T_a))*cos(wn*T_a*sqrt(1-ep^2))"
  Trigonometric Function1/1 -> Dot Product5/2  "cos(wn*T_a*sqrt(1-ep^2))"
  Ts/1 -> Dot Product/1
  Dot Product/1 -> Divide/2
  Dot Product3/1 -> Dot Product2/2  "-ep"
  Damping/1 -> Math Function1/1, Dot Product3/2, Dot Product/2  "ep"
  Constant/1 -> Divide/1
  Dot Product7/1 -> Dot Product6/1  "wn*T_a"
  Sample Time/1 -> Dot Product4/1, [B]  "T_a"
  Math Function1/1 -> Subtract/2  "ep^2"
  Dot Product1/1 -> Dot Product5/1  "-2*e^(cos(-ep*wn*T_a))"
  Constant2/1 -> Math Function1/2
  1/1 -> Subtract/1
  Constant1/1 -> Dot Product1/1
  Dot Product2/1 -> Dot Product4/2  "-ep*wn"
  [B] -> Dot Product7/2  "T_a"
  Dot Product6/1 -> Trigonometric Function1/1  "wn*T_a*sqrt(1-ep^2)"
  Dot Product4/1 -> Dot Product8/2, Math Function/1  "(-ep*wn*T_a)"
  Sqrt/1 -> Dot Product6/2  "sqrt(1-ep^2)"
  Subtract/1 -> Sqrt/1  "1-ep^2"
  Constant3/1 -> Dot Product8/1
  Dot Product8/1 -> Math Function2/1  "(-2*ep*wn*T_a)"
  Math Function2/1 -> Display1/1, P2/1  "exp(-2*ep*wn*T_a)"

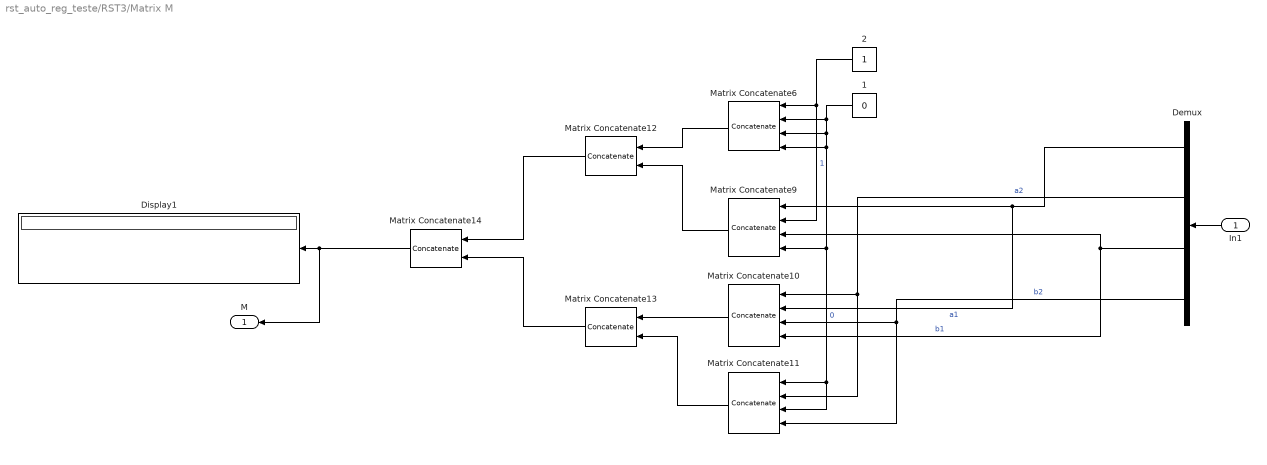
== system rst_auto_reg_teste/RST3/Matrix M ==
  In1 : Inport
  " 1" : Constant  Value=0
  2 : Constant
  Demux : Demux
  Display1 : Display
  Matrix Concatenate{6,9..11} (4 alike) : Concatenate  NumInputs=4  Mode=Multidimensional array  ConcatenateDimension=2
  Matrix Concatenate12 : Concatenate  Mode=Multidimensional array
  Matrix Concatenate13 : Concatenate  Mode=Multidimensional array
  Matrix Concatenate14 : Concatenate  Mode=Multidimensional array
  M : Outport
  wires:
  In1/1 -> Demux/1
  Demux/3 -> Matrix Concatenate9/3, Matrix Concatenate10/4  "b1"
  Matrix Concatenate14/1 -> M/1, Display1/1
  Demux/1 -> Matrix Concatenate10/2, Matrix Concatenate9/1  "a1"
  Demux/4 -> Matrix Concatenate11/4, Matrix Concatenate10/3  "b2"
  Demux/2 -> Matrix Concatenate11/2, Matrix Concatenate10/1  "a2"
  2/1 -> Matrix Concatenate9/2, Matrix Concatenate6/1  "1"
  " 1"/1 -> Matrix Concatenate6/3, Matrix Concatenate11/3, Matrix Concatenate11/1, Matrix Concatenate9/4, Matrix Concatenate6/4, Matrix Concatenate6/2  "0"
  Matrix Concatenate6/1 -> Matrix Concatenate12/1
  Matrix Concatenate9/1 -> Matrix Concatenate12/2
  Matrix Concatenate10/1 -> Matrix Concatenate13/1
  Matrix Concatenate11/1 -> Matrix Concatenate13/2
  Matrix Concatenate13/1 -> Matrix Concatenate14/2
  Matrix Concatenate12/1 -> Matrix Concatenate14/1

== system rst_auto_reg_teste/RST3/Matrix Q ==
  P1 : Inport
  P2 : Inport  Port=2
  Constant : Constant
  Constant1 : Constant  Value=0
  Display1 : Display
  Matrix Concatenate1 : Concatenate  Mode=Multidimensional array
  Matrix Concatenate2 : Concatenate  Mode=Multidimensional array
  Matrix Concatenate3 : Concatenate  Mode=Multidimensional array
  Q1 : Outport
  wires:
  Matrix Concatenate1/1 -> Matrix Concatenate2/1
  Matrix Concatenate2/1 -> Q1/1, Display1/1
  Matrix Concatenate3/1 -> Matrix Concatenate2/2
  P2/1 -> Matrix Concatenate3/1
  P1/1 -> Matrix Concatenate1/2
  Constant/1 -> Matrix Concatenate1/1
  Constant1/1 -> Matrix Concatenate3/2

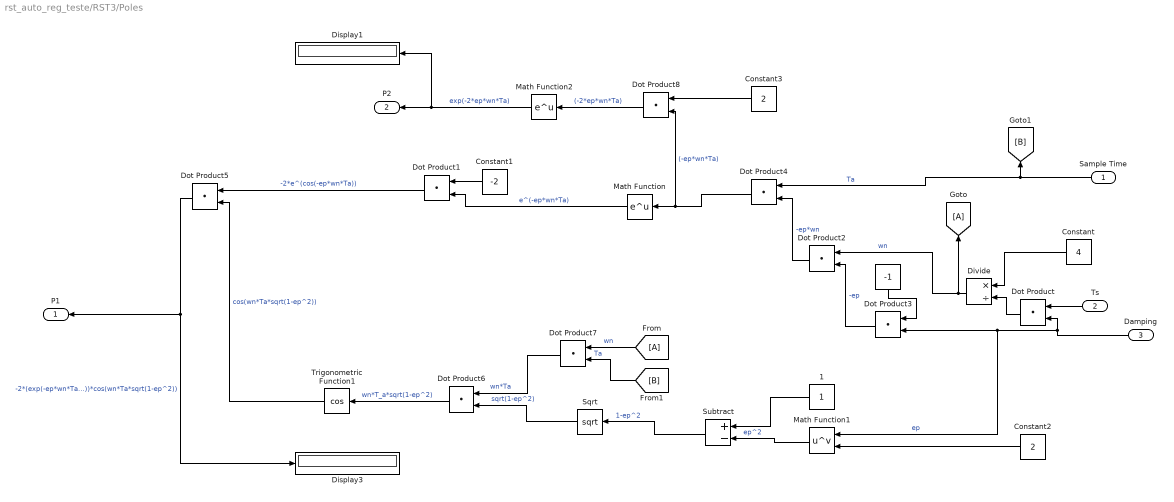
== system rst_auto_reg_teste/RST3/Poles ==
  Sample Time : Inport
  Ts : Inport  Port=2
  Damping : Inport  Port=3
  " " : Constant  Value=-1
  1 : Constant
  Constant : Constant  Value=4
  Constant1 : Constant  Value=-2
  Constant2 : Constant  Value=2
  Constant3 : Constant  Value=2
  Display1 : Display
  Display3 : Display
  Divide : Product  Inputs=*/
  Dot Product{,1..8} (9 alike) : DotProduct  InputSameDT=on  OutDataTypeStr=Inherit: Inherit via internal rule
  Math Function : Math  SaturateOnIntegerOverflow=on
  Math Function1 : Math  Operator=pow  SaturateOnIntegerOverflow=on
  Math Function2 : Math  SaturateOnIntegerOverflow=on
  Sqrt : Sqrt  SaturateOnIntegerOverflow=on
  Subtract : Sum  Inputs=+-
  Trigonometric Function1 : Trigonometry  Operator=cos
  P1 : Outport
  P2 : Outport  Port=2
  wires:
  Math Function/1 -> Dot Product1/2  "e^(-ep*wn*Ta)"
  Divide/1 -> [A], Dot Product2/1  "wn"
  [A] -> Dot Product7/1  "wn"
  " "/1 -> Dot Product3/1
  Dot Product5/1 -> P1/1, Display3/1  "-2*(exp(-ep*wn*Ta))*cos(wn*Ta*sqrt(1-ep^2))"
  Trigonometric Function1/1 -> Dot Product5/2  "cos(wn*Ta*sqrt(1-ep^2))"
  Ts/1 -> Dot Product/1
  Dot Product/1 -> Divide/2
  Dot Product3/1 -> Dot Product2/2  "-ep"
  Damping/1 -> Math Function1/1, Dot Product3/2, Dot Product/2  "ep"
  Constant/1 -> Divide/1
  Dot Product7/1 -> Dot Product6/1  "wn*Ta"
  Sample Time/1 -> Dot Product4/1, [B]  "Ta"
  Math Function1/1 -> Subtract/2  "ep^2"
  Dot Product1/1 -> Dot Product5/1  "-2*e^(cos(-ep*wn*Ta))"
  Constant2/1 -> Math Function1/2
  1/1 -> Subtract/1
  Constant1/1 -> Dot Product1/1
  Dot Product2/1 -> Dot Product4/2  "-ep*wn"
  [B] -> Dot Product7/2  "Ta"
  Dot Product6/1 -> Trigonometric Function1/1  "wn*T_a*sqrt(1-ep^2)"
  Dot Product4/1 -> Dot Product8/2, Math Function/1  "(-ep*wn*Ta)"
  Sqrt/1 -> Dot Product6/2  "sqrt(1-ep^2)"
  Subtract/1 -> Sqrt/1  "1-ep^2"
  Constant3/1 -> Dot Product8/1
  Dot Product8/1 -> Math Function2/1  "(-2*ep*wn*Ta)"
  Math Function2/1 -> Display1/1, P2/1  "exp(-2*ep*wn*Ta)"

== system rst_auto_reg_teste/Subsystem1/Vetor de Medidas  ==
  u : Inport
  y : Inport  Port=2
  Constant : Constant  Value=-1
  Delay{1..5} (5 alike) : Delay  DelayLength=1  InitialCondition=0  SampleTime=0.1
  Mux : Mux  Inputs=3
  Mux1 : Mux  Inputs=3
  Mux2 : Mux  Inputs=2
  Product : Product
  re : Outport
  wires:
  Delay4/1 -> Mux1/2, Delay5/1
  Delay5/1 -> Mux1/3
  Mux1/1 -> Mux2/2
  Mux/1 -> Mux2/1
  Mux2/1 -> re/1
  u/1 -> Mux1/1, Delay4/1
  Delay2/1 -> Mux/3
  y/1 -> Product/1
  Constant/1 -> Product/2
  Product/1 -> Delay1/1
  Delay3/1 -> Mux/2, Delay2/1
  Delay1/1 -> Mux/1, Delay3/1

== system rst_auto_reg_teste/Subsystem2/Vetor de Medidas  ==
  u : Inport
  y : Inport  Port=2
  Constant : Constant  Value=-1
  Delay{1..4} (4 alike) : Delay  DelayLength=1  InitialCondition=0  SampleTime=0.1
  Mux : Mux  Inputs=2
  Mux1 : Mux  Inputs=2
  Mux2 : Mux  Inputs=2
  Product : Product
  re : Outport
  wires:
  Delay4/1 -> Mux1/2  "u(t-2)"
  Mux1/1 -> Mux2/2
  Mux/1 -> Mux2/1
  Mux2/1 -> re/1
  u/1 -> Delay2/1
  y/1 -> Product/1
  Constant/1 -> Product/2
  Product/1 -> Delay1/1
  Delay3/1 -> Mux/2  "-y(t-2)"
  Delay1/1 -> Mux/1, Delay3/1  "-y(t-1)"
  Delay2/1 -> Mux1/1, Delay4/1  "u(t-1)"

== system rst_auto_reg_teste/Subsystem3/Vetor de Medidas  ==
  u : Inport
  y : Inport  Port=2
  Constant : Constant  Value=-1
  Delay{1..4} (4 alike) : Delay  DelayLength=1  InitialCondition=0  SampleTime=0.1
  Mux : Mux  Inputs=2
  Mux1 : Mux  Inputs=2
  Mux2 : Mux  Inputs=2
  Product : Product
  re : Outport
  wires:
  Delay4/1 -> Mux1/2  "u(t-2)"
  Mux1/1 -> Mux2/2
  Mux/1 -> Mux2/1
  Mux2/1 -> re/1
  u/1 -> Delay2/1
  y/1 -> Product/1
  Constant/1 -> Product/2
  Product/1 -> Delay1/1
  Delay3/1 -> Mux/2  "-y(t-2)"
  Delay1/1 -> Mux/1, Delay3/1  "-y(t-1)"
  Delay2/1 -> Mux1/1, Delay4/1  "u(t-1)"
